simulink model "lab2_simulink"  (R2023a)
settings: Solver=VariableStepAuto  StartTime=0.0  StopTime=10.0  RelTol=1e-3
libraries: simulink x2
settings Model: Creator=Dylan  LastModifiedBy=Dylan

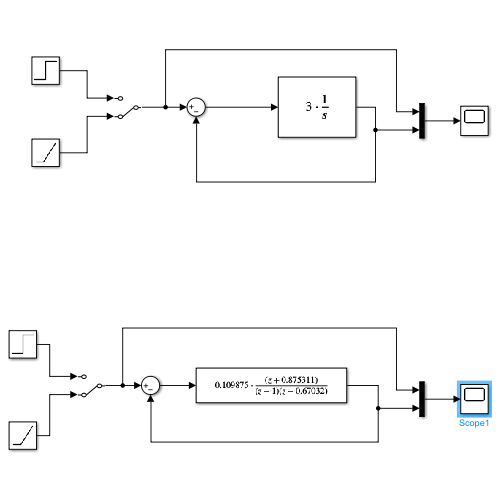
[thumbnail: Simulink's stored preview of the top-level diagram]
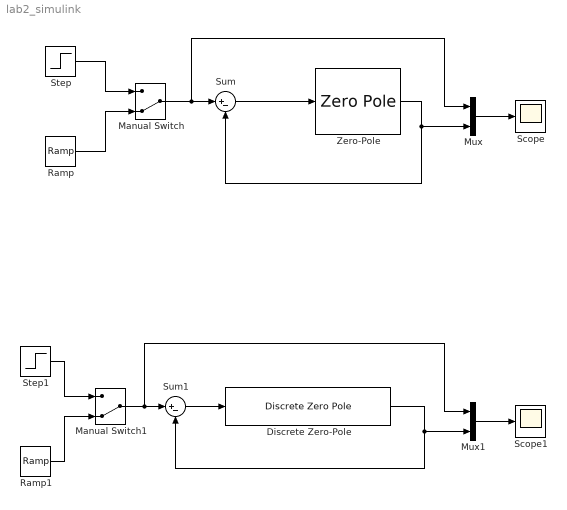
== system lab2_simulink ==
  Discrete Zero-Pole : DiscreteZeroPole  Zeros=[-0.875311]  Poles=[1 0.67032]  Gain=0.109875  SampleTime=-1
  Manual Switch : ManualSwitch  CurrentSetting=0
  Manual Switch1 : ManualSwitch  CurrentSetting=0
  Mux : Mux  Inputs=2
  Mux1 : Mux  Inputs=2
  Ramp : simulink/Sources/Ramp  slope=1  start=0  InitialOutput=0
  Ramp1 : simulink/Sources/Ramp  slope=1  start=0  InitialOutput=0
  Scope : Scope
  Scope1 : Scope
  Step : Step  Time=0  SampleTime=0
  Step1 : Step  Time=0  SampleTime=0
  Sum : Sum  Inputs=|+-
  Sum1 : Sum  Inputs=|+-
  Zero-Pole : ZeroPole  Zeros=[]  Poles=0  Gain=3
  wires:
  Step/1 -> Manual Switch/1
  Ramp/1 -> Manual Switch/2
  Manual Switch/1 -> Mux/1, Sum/1
  Zero-Pole/1 -> Sum/2, Mux/2
  Sum/1 -> Zero-Pole/1
  Mux/1 -> Scope/1
  Sum1/1 -> Discrete Zero-Pole/1
  Step1/1 -> Manual Switch1/1
  Ramp1/1 -> Manual Switch1/2
  Discrete Zero-Pole/1 -> Sum1/2, Mux1/2
  Mux1/1 -> Scope1/1
  Manual Switch1/1 -> Sum1/1, Mux1/1
